simulink model "STDiscovery2016a"  (R2017b)
settings: Solver=FixedStepAuto  StartTime=0.0  StopTime=10  FixedStep=Abtastzeit  RelTol=1e-3
PreLoadFcn:
  | waijung.modelPreload; % Required for working with Waijung Blockset. Do not remove.
model workspace (MAT data in the model file):
  Abtastzeit = 0.01
  Servo_IN_min = 0.894
  SimulationDutyCycle = 27
undefined symbols (not defined in the file): HSEOSC, Link, LQFP176, ST, STM32F417IG
libraries: stm32f4_io_lib x15, simulink x10, simulink_extras x8, stm32f4_adc_lib x7, powerlib_meascontrol x3, stm32f4_device_config_lib x1
(part 4 of 5)

== system STDiscovery2016a/Debug/Subsystem2 ==
  In1 : Inport
  In2 : Inport  Port=2
  In3 : Inport  Port=3
  Enable : EnablePort
  Data Type Conversion : DataTypeConversion
  Data Type Conversion1 : DataTypeConversion
  Data Type Conversion2 : DataTypeConversion
  UART Tx : S-Function  Priority=1  FunctionName=stm32f4_usart  Parameters=configuration,uartmodule,transfer,baudrate,inputtype,outputtype,confstr,binheaderarray,binterminatorarray,asciiheader,asciiterminator,bindatalength,packetmode,varname,sampletime,sampletimestr,blockid  SFunctionDeploymentMode=off  EnableBusSupport=off  mask(stm32f4_usart){configuration=Tx, uartmodule=3, baudrate=115200, databits=8, parity=No, stopbit=1, remaptxpin=Not used, remaprxpin=Not used, flowcontrol=None, remapctspin=Not used, remaprtspin=Not used, advanceoptions=off, rxbuffersize=512, txbuffersize=512, transfer=Blocking, packetmode=Ascii, binheader='7E 7E', binterminator='03 03', porttype_double=1, porttype_single=0, porttype_int8=1, porttype_uint8=0, porttype_int16=0, porttype_uint16=0, porttype_int32=0, porttype_uint32=0, asciiformat='READ Servo:%f sec, %f Prozent, %f Hz\n', rx_asciiterminator=CRLF (0x0D 0x0A - "\r\n"), tx_asciiterminator=CRLF (0x0D 0x0A - "\r\n"), storagename=S, varname=, inputtype=[3  1 1 1], outputtype=[0], binheaderarray=[0], binterminatorarray=[0], bindatalength=0, asciiheader='READ Servo:%f sec, %f Prozent, %f Hz\n\r\n', asciiterminator=[2 13 10], sampletime=0.1, sampletimestr=-1, blockid=DebugSubsystem2UARTTx, confstr=[ "dummy", "0", "*", "*", "0", "*", "*", "0", "*", "*", "0", "*", "*", "1", "4", "3", "1", "4", "1", "512", "512", "1", "3", "115200", "8", "No", "1", "None", "USART3"], lastmodule=1}
      mask prompts: uartmodule "UART Module"; baudrate "Baud rate (bps)"; databits "Data bits"; stopbit "Stop bit"; remaptxpin "Tx Pin"; remaprxpin "Rx Pin"; flowcontrol "Hardware flow control"; remapctspin "HW Flow control, CTS Pin"; remaprtspin "HW Flow control, RTS Pin"; advanceoptions "Advance options"; rxbuffersize "Rx buffer size (bytes)"; txbuffersize "Tx buffer size (bytes)"; packetmode "Packet mode"; binheader "Binary header (example: '7E 7E')"; binterminator "Binary terminator (example: '03 03')"; porttype_double "Number of data port, type DOUBLE"; porttype_single "Number of data port, type SINGLE"; porttype_int8 "Number of data port, type INT8"; porttype_uint8 "Number of data port, type UINT8"; porttype_int16 "Number of data port, type INT16"; porttype_uint16 "Number of data port, type UINT16"; porttype_int32 "Number of data port, type INT32"; porttype_uint32 "Number of data port, type UINT32"; asciiformat "Ascii format"; rx_asciiterminator "End of packet"; tx_asciiterminator "End of packet"; storagename "Buffer"; varname "Var name"; inputtype "Input data type"; outputtype "Output data type"; binheaderarray "Binary header"; binterminatorarray "Binary terminator"; bindatalength "Binary data length"; asciiheader "Ascii header (printf format)"; asciiterminator "Ascii terminator"; sampletime "Sample time (sec)"; sampletimestr "Compiled sample time (sec) in string"; confstr "Configuration string"; lastmodule "Last module selected"
      mask help:
      | Data type for Ascii format
      | %u, %i, %d, %o, %x: uint32
      | %e, %g, %f: single
      | %c: int8
      mask init:
      | stm32f4_usart_callback('init');
      mask Help: web(fullfile(waijungdocroot,'stm32f4_usart_tx.htm'), '-browser')
      mask TypeOptions configuration: Setup | Tx | Rx
      mask Callback configuration: stm32f4_usart_callback('configuration');
      mask TypeOptions uartmodule: 1 | 2 | 3 | 4 | 5 | 6
      mask Callback uartmodule: stm32f4_usart_callback('uartmodule');
      mask Callback baudrate: stm32f4_usart_callback('baudrate');
      mask TypeOptions databits: 8
      mask TypeOptions parity: No | Odd | Even
      mask TypeOptions stopbit: 0.5 | 1 | 1.5 | 2
      mask TypeOptions remaptxpin: Not used | A9 | B6
      mask TypeOptions remaprxpin: Not used | A10 | B7
      mask TypeOptions flowcontrol: None | RTS | CTS | RTS/CTS
      mask Callback flowcontrol: stm32f4_usart_callback('flowcontrol');
      mask TypeOptions remapctspin: Not used | A11
      mask TypeOptions remaprtspin: Not used | A12
      mask Callback advanceoptions: stm32f4_usart_callback('advanceoptions');
      mask TypeOptions rxbuffersize: 16 | 32 | 64 | 128 | 256 | 512 | 1024 | 2048
      mask TypeOptions txbuffersize: 16 | 32 | 64 | 128 | 256 | 512 | 1024 | 2048
      mask TypeOptions transfer: Blocking | Non-Blocking
      mask Callback transfer: stm32f4_usart_callback('transfer');
      mask TypeOptions packetmode: Ascii | Binary | String Buffer
      mask Callback packetmode: stm32f4_usart_callback('packetmode');
      mask Callback binheader: stm32f4_usart_callback('binheader');
      mask Callback binterminator: stm32f4_usart_callback('binterminator');
      mask Callback porttype_double: stm32f4_usart_callback('porttype');
      mask Callback porttype_single: stm32f4_usart_callback('porttype');
      mask Callback porttype_int8: stm32f4_usart_callback('porttype');
      mask Callback porttype_uint8: stm32f4_usart_callback('porttype');
      mask Callback porttype_int16: stm32f4_usart_callback('porttype');
      mask Callback porttype_uint16: stm32f4_usart_callback('porttype');
      mask Callback porttype_int32: stm32f4_usart_callback('porttype');
      mask Callback porttype_uint32: stm32f4_usart_callback('porttype');
      mask Callback asciiformat: stm32f4_usart_callback('asciiformat');
      mask TypeOptions rx_asciiterminator: CR (0x0D - "\r") | LF (0x0A - "\n") | CRLF (0x0D 0x0A - "\r\n")
      mask Callback rx_asciiterminator: stm32f4_usart_callback('rx_asciiterminator');
      mask TypeOptions tx_asciiterminator: CR (0x0D - "\r") | LF (0x0A - "\n") | CRLF (0x0D 0x0A - "\r\n") | None
      mask Callback tx_asciiterminator: stm32f4_usart_callback('tx_asciiterminator');
      mask TypeOptions storagename: <Please insert a storage name> | S
      mask Callback storagename: stm32f4_usart_callback('storagename');
      mask Callback varname: stm32f4_usart_callback('varname');
      mask Callback sampletime: stm32f4_usart_callback('sampletime');
      mask Callback sampletimestr: stm32f4_usart_callback('sampletimestr');
      mask Callback blockid: stm32f4_usart_callback('blockid');
      mask Display: text(0.95, 0.5, 'Module: USART3_Tx\nPacket: Ascii\nTransfer: Blocking\nTs (sec): -1','ver','middle','hor','right'); port_label('input', 1,'single'); port_label('input', 2,'single'); port_label('input', 3,'single');
  wires:
  Data Type Conversion/1 -> UART Tx/1
  In1/1 -> Data Type Conversion/1
  In3/1 -> Data Type Conversion2/1
  In2/1 -> Data Type Conversion1/1
  Data Type Conversion1/1 -> UART Tx/2
  Data Type Conversion2/1 -> UART Tx/3

== system STDiscovery2016a/Debug/Subsystem3 ==
  In1 : Inport
  In2 : Inport  Port=2
  In3 : Inport  Port=3
  Enable : EnablePort
  Data Type Conversion : DataTypeConversion
  Data Type Conversion1 : DataTypeConversion
  Data Type Conversion2 : DataTypeConversion
  UART Tx1 : S-Function  Priority=1  FunctionName=stm32f4_usart  Parameters=configuration,uartmodule,transfer,baudrate,inputtype,outputtype,confstr,binheaderarray,binterminatorarray,asciiheader,asciiterminator,bindatalength,packetmode,varname,sampletime,sampletimestr,blockid  SFunctionDeploymentMode=off  EnableBusSupport=off  mask(stm32f4_usart){configuration=Tx, uartmodule=3, baudrate=115200, databits=8, parity=No, stopbit=1, remaptxpin=Not used, remaprxpin=Not used, flowcontrol=None, remapctspin=Not used, remaprtspin=Not used, advanceoptions=off, rxbuffersize=512, txbuffersize=512, transfer=Blocking, packetmode=Ascii, binheader='7E 7E', binterminator='03 03', porttype_double=1, porttype_single=0, porttype_int8=1, porttype_uint8=0, porttype_int16=0, porttype_uint16=0, porttype_int32=0, porttype_uint32=0, asciiformat='Antwort von ST:    TEST1: %f   , TEST2: %f   ,TEST2:  %f', rx_asciiterminator=CRLF (0x0D 0x0A - "\r\n"), tx_asciiterminator=CRLF (0x0D 0x0A - "\r\n"), storagename=S, varname=, inputtype=[3  1 1 1], outputtype=[0], binheaderarray=[0], binterminatorarray=[0], bindatalength=0, asciiheader='Antwort von ST:    TEST1: %f   , TEST2: %f   ,TEST2:  %f\r\n', asciiterminator=[2 13 10], sampletime=0.1, sampletimestr=0.1, blockid=DebugSubsystem3UARTTx1, confstr=[ "dummy", "0", "*", "*", "0", "*", "*", "0", "*", "*", "0", "*", "*", "1", "4", "3", "1", "4", "1", "512", "512", "1", "3", "115200", "8", "No", "1", "None", "USART3"], lastmodule=1}
      mask prompts: uartmodule "UART Module"; baudrate "Baud rate (bps)"; databits "Data bits"; stopbit "Stop bit"; remaptxpin "Tx Pin"; remaprxpin "Rx Pin"; flowcontrol "Hardware flow control"; remapctspin "HW Flow control, CTS Pin"; remaprtspin "HW Flow control, RTS Pin"; advanceoptions "Advance options"; rxbuffersize "Rx buffer size (bytes)"; txbuffersize "Tx buffer size (bytes)"; packetmode "Packet mode"; binheader "Binary header (example: '7E 7E')"; binterminator "Binary terminator (example: '03 03')"; porttype_double "Number of data port, type DOUBLE"; porttype_single "Number of data port, type SINGLE"; porttype_int8 "Number of data port, type INT8"; porttype_uint8 "Number of data port, type UINT8"; porttype_int16 "Number of data port, type INT16"; porttype_uint16 "Number of data port, type UINT16"; porttype_int32 "Number of data port, type INT32"; porttype_uint32 "Number of data port, type UINT32"; asciiformat "Ascii format"; rx_asciiterminator "End of packet"; tx_asciiterminator "End of packet"; storagename "Buffer"; varname "Var name"; inputtype "Input data type"; outputtype "Output data type"; binheaderarray "Binary header"; binterminatorarray "Binary terminator"; bindatalength "Binary data length"; asciiheader "Ascii header (printf format)"; asciiterminator "Ascii terminator"; sampletime "Sample time (sec)"; sampletimestr "Compiled sample time (sec) in string"; confstr "Configuration string"; lastmodule "Last module selected"
      mask help:
      | Data type for Ascii format
      | %u, %i, %d, %o, %x: uint32
      | %e, %g, %f: single
      | %c: int8
      mask init:
      | stm32f4_usart_callback('init');
      mask Help: web(fullfile(waijungdocroot,'stm32f4_usart_tx.htm'), '-browser')
      mask TypeOptions configuration: Setup | Tx | Rx
      mask Callback configuration: stm32f4_usart_callback('configuration');
      mask TypeOptions uartmodule: 1 | 2 | 3 | 4 | 5 | 6
      mask Callback uartmodule: stm32f4_usart_callback('uartmodule');
      mask Callback baudrate: stm32f4_usart_callback('baudrate');
      mask TypeOptions databits: 8
      mask TypeOptions parity: No | Odd | Even
      mask TypeOptions stopbit: 0.5 | 1 | 1.5 | 2
      mask TypeOptions remaptxpin: Not used | A9 | B6
      mask TypeOptions remaprxpin: Not used | A10 | B7
      mask TypeOptions flowcontrol: None | RTS | CTS | RTS/CTS
      mask Callback flowcontrol: stm32f4_usart_callback('flowcontrol');
      mask TypeOptions remapctspin: Not used | A11
      mask TypeOptions remaprtspin: Not used | A12
      mask Callback advanceoptions: stm32f4_usart_callback('advanceoptions');
      mask TypeOptions rxbuffersize: 16 | 32 | 64 | 128 | 256 | 512 | 1024 | 2048
      mask TypeOptions txbuffersize: 16 | 32 | 64 | 128 | 256 | 512 | 1024 | 2048
      mask TypeOptions transfer: Blocking | Non-Blocking
      mask Callback transfer: stm32f4_usart_callback('transfer');
      mask TypeOptions packetmode: Ascii | Binary | String Buffer
      mask Callback packetmode: stm32f4_usart_callback('packetmode');
      mask Callback binheader: stm32f4_usart_callback('binheader');
      mask Callback binterminator: stm32f4_usart_callback('binterminator');
      mask Callback porttype_double: stm32f4_usart_callback('porttype');
      mask Callback porttype_single: stm32f4_usart_callback('porttype');
      mask Callback porttype_int8: stm32f4_usart_callback('porttype');
      mask Callback porttype_uint8: stm32f4_usart_callback('porttype');
      mask Callback porttype_int16: stm32f4_usart_callback('porttype');
      mask Callback porttype_uint16: stm32f4_usart_callback('porttype');
      mask Callback porttype_int32: stm32f4_usart_callback('porttype');
      mask Callback porttype_uint32: stm32f4_usart_callback('porttype');
      mask Callback asciiformat: stm32f4_usart_callback('asciiformat');
      mask TypeOptions rx_asciiterminator: CR (0x0D - "\r") | LF (0x0A - "\n") | CRLF (0x0D 0x0A - "\r\n")
      mask Callback rx_asciiterminator: stm32f4_usart_callback('rx_asciiterminator');
      mask TypeOptions tx_asciiterminator: CR (0x0D - "\r") | LF (0x0A - "\n") | CRLF (0x0D 0x0A - "\r\n") | None
      mask Callback tx_asciiterminator: stm32f4_usart_callback('tx_asciiterminator');
      mask TypeOptions storagename: <Please insert a storage name> | S
      mask Callback storagename: stm32f4_usart_callback('storagename');
      mask Callback varname: stm32f4_usart_callback('varname');
      mask Callback sampletime: stm32f4_usart_callback('sampletime');
      mask Callback sampletimestr: stm32f4_usart_callback('sampletimestr');
      mask Callback blockid: stm32f4_usart_callback('blockid');
      mask Display: text(0.95, 0.5, 'Module: USART3_Tx\nPacket: Ascii\nTransfer: Blocking\nTs (sec): 0.1','ver','middle','hor','right'); port_label('input', 1,'single'); port_label('input', 2,'single'); port_label('input', 3,'single');
  wires:
  Data Type Conversion/1 -> UART Tx1/1
  In1/1 -> Data Type Conversion/1
  Data Type Conversion2/1 -> UART Tx1/3
  Data Type Conversion1/1 -> UART Tx1/2
  In2/1 -> Data Type Conversion1/1
  In3/1 -> Data Type Conversion2/1

== system STDiscovery2016a/Power Distribution Unit/Sicherung Akku ==
  note: Analoger Eingang
      | (Stromverbrauch)
  note: Digitaler Eingang
      | Sicherung zurücksetzen
  Logical Operator1 : Logic  Operator=NOT  AllPortsSameDT=off  OutDataTypeStr=boolean
  Minimaler Wert : Constant  Value=6.6
  Restspannung Akku : stm32f4_adc_lib/Regular ADC  adcmodule=1  outputdatatype=Double  prescaler=2  prescalerstr=ADC_Prescaler_Div2  chsamplingtime=Auto  chsamplingtimestr=ADC_SampleTime_480Cycles  read_an0=off  read_an1=off  read_an2=off  read_an3=off  read_an4=off  read_an5=off  read_an6=on  read_an7=off  read_an8=off  read_an9=off  read_an10=off  read_an11=off  read_an12=off  read_an13=off  read_an14=off  read_an15=off  read_an16=off  read_an17=off  read_an18=off  pinstr=GPIO_Pin_6  usedpinarray="[0  0  0  0  0  0  1  0  0  0  0  0  0  0  0  0  0  0  0]"  usedportidarray=[0]  usedpinidarray=[6]  usedpinidcount=1  sampletime=Abtastzeit  blockid=PowerDistributionUnitSicherungAkkuRestspannungAkku  enablecustomportlabel=off  cinputportlabel=0  coutputportlabel=Out1, Out2
      settings: SourceProductName=Waijung Blockset
  Sicherung ausloesen : stm32f4_io_lib/Digital Output  use_bitband=on  port=D  speed=100  porttype=Push Pull  porttypestr=PP  use_pin0=off  use_pin1=off  use_pin2=off  use_pin3=off  use_pin4=off  use_pin5=off  use_pin6=on  use_pin7=off  use_pin8=off  use_pin9=off  use_pin10=off  use_pin11=off  use_pin12=off  use_pin13=off  use_pin14=off  use_pin15=off  pinstr=GPIO_Pin_6  usedpinarray="[0  0  0  0  0  0  1  0  0  0  0  0  0  0  0  0]"  bitbandingstr="#define PowerDistributionUnitSicherungAkkuSicherungausloesen_D6 Peripheral_BB(GPIOD->ODR, 6)  /* Output pin */"  sampletime=Abtastzeit  sampletimestr=-1  blockid=PowerDistributionUnitSicherungAkkuSicherungausloesen  enablecustomportlabel=off  globalinit=off  cinputportlabel=In1, In2  coutputportlabel=0
      settings: SourceProductName=Waijung Blockset
  Sicherung gefallen : simulink_extras/Flip Flops/S-R Flip-Flop  initial_condition=0
  Sicherung nicht wieder einschalten wenn maximaler wert noch ueberschritten ist : Logic  AllPortsSameDT=off  OutDataTypeStr=boolean
  Sicherungen Ruecksetzen (User Button 1) (Loetbruecke bei sb20 noetig laut Manual) : stm32f4_io_lib/Digital Input  port=A  speed=100  porttype=None  porttypestr=NOPULL  use_pin0=on  use_pin1=off  use_pin2=off  use_pin3=off  use_pin4=off  use_pin5=off  use_pin6=off  use_pin7=off  use_pin8=off  use_pin9=off  use_pin10=off  use_pin11=off  use_pin12=off  use_pin13=off  use_pin14=off  use_pin15=off  pinstr=GPIO_Pin_0  usedpinarray="[1  0  0  0  0  0  0  0  0  0  0  0  0  0  0  0]"  bitbandingstr="#define PowerDistributionUnitSicherungAkkuSicherungenRuecksetzenUserButton1Loetbrueckebeisb20noetiglautManual_A0 Peripheral_BB(GPIOA->IDR, 0)  /* Output pin */"  sampletime=Abtastzeit  sampletimestr=-1  blockid=PowerDistributionUnitSicherungAkkuSicherungenRuecksetzenUserButton1Loetbrueckebeisb20noetiglautManual  enablecustomportlabel=off  glabalinit=off  cinputportlabel=In1, In2  coutputportlabel=Out1, Out2
      settings: SourceProductName=Waijung Blockset
  Terminator : Terminator
  Umwandlung in Range nach 5V : Gain  Gain=5/4095  ParamDataTypeStr=double  OutDataTypeStr=double
  Wurde minimaler Wert unterschritten? : RelationalOperator  Operator=>  OutDataTypeStr=boolean  RndMeth=Nearest
  wires:
  Umwandlung in Range nach 5V/1 -> Wurde minimaler Wert unterschritten?/2
  Minimaler Wert/1 -> Wurde minimaler Wert unterschritten?/1
  Wurde minimaler Wert unterschritten?/1 -> Logical Operator1/1, Sicherung gefallen/1
  Sicherung gefallen/1 -> Sicherung ausloesen/1
  Restspannung Akku/1 -> Umwandlung in Range nach 5V/1
  Sicherungen Ruecksetzen (User Button 1) (Loetbruecke bei sb20 noetig laut Manual)/1 -> Sicherung nicht wieder einschalten wenn maximaler wert noch ueberschritten ist/2
  Sicherung nicht wieder einschalten wenn maximaler wert noch ueberschritten ist/1 -> Sicherung gefallen/2
  Logical Operator1/1 -> Sicherung nicht wieder einschalten wenn maximaler wert noch ueberschritten ist/1
  Sicherung gefallen/2 -> Terminator/1

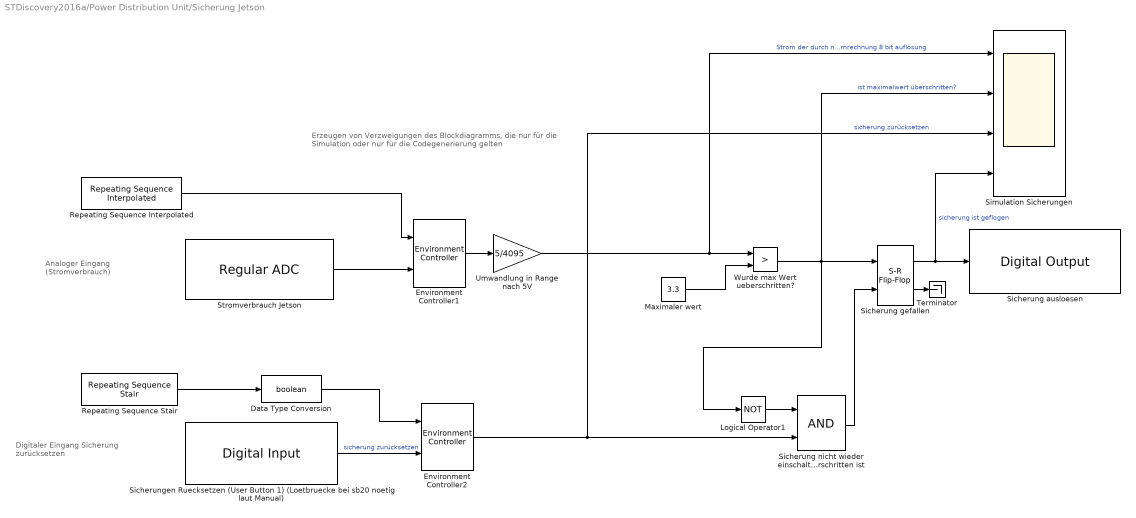
== system STDiscovery2016a/Power Distribution Unit/Sicherung Jetson ==
  note: Analoger Eingang
      | (Stromverbrauch)
  note: Erzeugen von Verzweigungen des Blockdiagramms,
      | die nur für die Simulation oder nur für die Codegenerierung gelten
  note: Digitaler Eingang
      | Sicherung zurücksetzen
  Data Type Conversion : DataTypeConversion  OutDataTypeStr=boolean
  Environment Controller1 : simulink/Signal Routing/Environment Controller
      settings: SourceProductName=Simulink  SourceProductBaseCode=SL
  Environment Controller2 : simulink/Signal Routing/Environment Controller
      settings: SourceProductName=Simulink  SourceProductBaseCode=SL
  Logical Operator1 : Logic  Operator=NOT  AllPortsSameDT=off  OutDataTypeStr=boolean
  Maximaler wert : Constant  Value=3.3
  Repeating Sequence Interpolated : simulink/Sources/Repeating Sequence Interpolated  OutValues=[2000 3000 2000].'  TimeValues=[0 5 10].'  LookUpMeth=Interpolation-Use End Values  tsamp=0.01  OutMin=[]  OutMax=[]  OutDataTypeStr=double  OutputDataTypeScalingMode=double  OutDataType=fixdt(0,8)  OutScaling=2^-10
  Repeating Sequence Stair : simulink/Sources/Repeating Sequence Stair  OutValues=[0 0 0 0 1 0 0 1 0 0].'  tsamp=1  OutMin=[]  OutMax=[]  OutDataTypeStr=double  OutputDataTypeScalingMode=double  OutDataType=fixdt(0,8)  ConRadixGroup=Best Precision: Vector-wise  OutScaling=2^-12
  Sicherung ausloesen : stm32f4_io_lib/Digital Output  use_bitband=on  port=D  speed=100  porttype=Push Pull  porttypestr=PP  use_pin0=on  use_pin1=off  use_pin2=off  use_pin3=off  use_pin4=off  use_pin5=off  use_pin6=off  use_pin7=off  use_pin8=off  use_pin9=off  use_pin10=off  use_pin11=off  use_pin12=off  use_pin13=off  use_pin14=off  use_pin15=off  pinstr=GPIO_Pin_0  usedpinarray="[1  0  0  0  0  0  0  0  0  0  0  0  0  0  0  0]"  bitbandingstr="#define PowerDistributionUnitSicherungJetsonSicherungausloesen_D0 Peripheral_BB(GPIOD->ODR, 0)  /* Output pin */"  sampletime=Abtastzeit  sampletimestr=-1  blockid=PowerDistributionUnitSicherungJetsonSicherungausloesen  enablecustomportlabel=off  globalinit=off  cinputportlabel=In1, In2  coutputportlabel=0
      settings: SourceProductName=Waijung Blockset
  Sicherung gefallen : simulink_extras/Flip Flops/S-R Flip-Flop  initial_condition=0
  Sicherung nicht wieder einschalten wenn maximaler wert noch ueberschritten ist : Logic  AllPortsSameDT=off  OutDataTypeStr=boolean
  Sicherungen Ruecksetzen (User Button 1) (Loetbruecke bei sb20 noetig laut Manual) : stm32f4_io_lib/Digital Input  port=A  speed=100  porttype=None  porttypestr=NOPULL  use_pin0=on  use_pin1=off  use_pin2=off  use_pin3=off  use_pin4=off  use_pin5=off  use_pin6=off  use_pin7=off  use_pin8=off  use_pin9=off  use_pin10=off  use_pin11=off  use_pin12=off  use_pin13=off  use_pin14=off  use_pin15=off  pinstr=GPIO_Pin_0  usedpinarray="[1  0  0  0  0  0  0  0  0  0  0  0  0  0  0  0]"  bitbandingstr="#define PowerDistributionUnitSicherungJetsonSicherungenRuecksetzenUserButton1Loetbrueckebeisb20noetiglautManual_A0 Peripheral_BB(GPIOA->IDR, 0)  /* Output pin */"  sampletime=Abtastzeit  sampletimestr=-1  blockid=PowerDistributionUnitSicherungJetsonSicherungenRuecksetzenUserButton1Loetbrueckebeisb20noetiglautManual  enablecustomportlabel=off  glabalinit=off  cinputportlabel=In1, In2  coutputportlabel=Out1, Out2
      settings: SourceProductName=Waijung Blockset
  Simulation Sicherungen : Scope  NumInputPorts=4
  Stromverbrauch Jetson : stm32f4_adc_lib/Regular ADC  adcmodule=1  outputdatatype=Double  prescaler=2  prescalerstr=ADC_Prescaler_Div2  chsamplingtime=Auto  chsamplingtimestr=ADC_SampleTime_480Cycles  read_an0=off  read_an1=on  read_an2=off  read_an3=off  read_an4=off  read_an5=off  read_an6=off  read_an7=off  read_an8=off  read_an9=off  read_an10=off  read_an11=off  read_an12=off  read_an13=off  read_an14=off  read_an15=off  read_an16=off  read_an17=off  read_an18=off  pinstr=GPIO_Pin_1  usedpinarray="[0  1  0  0  0  0  0  0  0  0  0  0  0  0  0  0  0  0  0]"  usedportidarray=[0]  usedpinidarray=[1]  usedpinidcount=1  sampletime=Abtastzeit  blockid=PowerDistributionUnitSicherungJetsonStromverbrauchJetson  enablecustomportlabel=off  cinputportlabel=0  coutputportlabel=Out1, Out2
      settings: SourceProductName=Waijung Blockset
  Terminator : Terminator
  Umwandlung in Range nach 5V : Gain  Gain=5/4095  ParamDataTypeStr=double  OutDataTypeStr=double
  Wurde max Wert ueberschritten? : RelationalOperator  Operator=>  OutDataTypeStr=boolean  RndMeth=Nearest
  wires:
  Umwandlung in Range nach 5V/1 -> Simulation Sicherungen/1, Wurde max Wert ueberschritten?/1  "Strom der durch ne spannujng ausgedrückt wird nach der umrechnung 8 bit auflösung"
  Maximaler wert/1 -> Wurde max Wert ueberschritten?/2
  Wurde max Wert ueberschritten?/1 -> Logical Operator1/1, Simulation Sicherungen/2, Sicherung gefallen/1  "ist maximalwert überschritten?"
  Environment Controller2/1 -> Sicherung nicht wieder einschalten wenn maximaler wert noch ueberschritten ist/2, Simulation Sicherungen/3  "sicherung zurücksetzen"
  Sicherung gefallen/1 -> Simulation Sicherungen/4, Sicherung ausloesen/1  "sicherung ist geflogen"
  Stromverbrauch Jetson/1 -> Environment Controller1/2
  Repeating Sequence Stair/1 -> Data Type Conversion/1
  Repeating Sequence Interpolated/1 -> Environment Controller1/1
  Sicherung nicht wieder einschalten wenn maximaler wert noch ueberschritten ist/1 -> Sicherung gefallen/2
  Logical Operator1/1 -> Sicherung nicht wieder einschalten wenn maximaler wert noch ueberschritten ist/1
  Data Type Conversion/1 -> Environment Controller2/1
  Environment Controller1/1 -> Umwandlung in Range nach 5V/1
  Sicherungen Ruecksetzen (User Button 1) (Loetbruecke bei sb20 noetig laut Manual)/1 -> Environment Controller2/2  "sicherung zurücksetzen"
  Sicherung gefallen/2 -> Terminator/1

== system STDiscovery2016a/Power Distribution Unit/Sicherung Motor ==
  note: Analoger Eingang
      | (Stromverbrauch)
  note: Digitaler Eingang
      | Sicherung zurücksetzen
  Logical Operator1 : Logic  Operator=NOT  AllPortsSameDT=off  OutDataTypeStr=boolean
  Maximaler wert : Constant  Value=3.3
  Sicherung ausloesen : stm32f4_io_lib/Digital Output  use_bitband=on  port=D  speed=100  porttype=Push Pull  porttypestr=PP  use_pin0=off  use_pin1=off  use_pin2=off  use_pin3=on  use_pin4=off  use_pin5=off  use_pin6=off  use_pin7=off  use_pin8=off  use_pin9=off  use_pin10=off  use_pin11=off  use_pin12=off  use_pin13=off  use_pin14=off  use_pin15=off  pinstr=GPIO_Pin_3  usedpinarray="[0  0  0  1  0  0  0  0  0  0  0  0  0  0  0  0]"  bitbandingstr="#define PowerDistributionUnitSicherungMotorSicherungausloesen_D3 Peripheral_BB(GPIOD->ODR, 3)  /* Output pin */"  sampletime=Abtastzeit  sampletimestr=-1  blockid=PowerDistributionUnitSicherungMotorSicherungausloesen  enablecustomportlabel=off  globalinit=off  cinputportlabel=In1, In2  coutputportlabel=0
      settings: SourceProductName=Waijung Blockset
  Sicherung gefallen : simulink_extras/Flip Flops/S-R Flip-Flop  initial_condition=0
  Sicherung nicht wieder einschalten wenn maximaler wert noch ueberschritten ist : Logic  AllPortsSameDT=off  OutDataTypeStr=boolean
  Sicherungen Ruecksetzen (User Button 1) (Loetbruecke bei sb20 noetig laut Manual) : stm32f4_io_lib/Digital Input  port=A  speed=100  porttype=None  porttypestr=NOPULL  use_pin0=on  use_pin1=off  use_pin2=off  use_pin3=off  use_pin4=off  use_pin5=off  use_pin6=off  use_pin7=off  use_pin8=off  use_pin9=off  use_pin10=off  use_pin11=off  use_pin12=off  use_pin13=off  use_pin14=off  use_pin15=off  pinstr=GPIO_Pin_0  usedpinarray="[1  0  0  0  0  0  0  0  0  0  0  0  0  0  0  0]"  bitbandingstr="#define PowerDistributionUnitSicherungMotorSicherungenRuecksetzenUserButton1Loetbrueckebeisb20noetiglautManual_A0 Peripheral_BB(GPIOA->IDR, 0)  /* Output pin */"  sampletime=Abtastzeit  sampletimestr=-1  blockid=PowerDistributionUnitSicherungMotorSicherungenRuecksetzenUserButton1Loetbrueckebeisb20noetiglautManual  enablecustomportlabel=off  glabalinit=off  cinputportlabel=In1, In2  coutputportlabel=Out1, Out2
      settings: SourceProductName=Waijung Blockset
  Stromverbrauch Motor : stm32f4_adc_lib/Regular ADC  adcmodule=1  outputdatatype=Double  prescaler=2  prescalerstr=ADC_Prescaler_Div2  chsamplingtime=Auto  chsamplingtimestr=ADC_SampleTime_480Cycles  read_an0=off  read_an1=off  read_an2=off  read_an3=on  read_an4=off  read_an5=off  read_an6=off  read_an7=off  read_an8=off  read_an9=off  read_an10=off  read_an11=off  read_an12=off  read_an13=off  read_an14=off  read_an15=off  read_an16=off  read_an17=off  read_an18=off  pinstr=GPIO_Pin_3  usedpinarray="[0  0  0  1  0  0  0  0  0  0  0  0  0  0  0  0  0  0  0]"  usedportidarray=[0]  usedpinidarray=[3]  usedpinidcount=1  sampletime=Abtastzeit  blockid=PowerDistributionUnitSicherungMotorStromverbrauchMotor  enablecustomportlabel=off  cinputportlabel=0  coutputportlabel=Out1, Out2
      settings: SourceProductName=Waijung Blockset
  Terminator : Terminator
  Umwandlung in Range nach 5V : Gain  Gain=5/4095  ParamDataTypeStr=double  OutDataTypeStr=double
  Wurde max Wert überschritten? : RelationalOperator  Operator=>  OutDataTypeStr=boolean  RndMeth=Nearest
  wires:
  Umwandlung in Range nach 5V/1 -> Wurde max Wert überschritten?/1
  Maximaler wert/1 -> Wurde max Wert überschritten?/2
  Wurde max Wert überschritten?/1 -> Logical Operator1/1, Sicherung gefallen/1
  Sicherung gefallen/1 -> Sicherung ausloesen/1
  Stromverbrauch Motor/1 -> Umwandlung in Range nach 5V/1
  Sicherungen Ruecksetzen (User Button 1) (Loetbruecke bei sb20 noetig laut Manual)/1 -> Sicherung nicht wieder einschalten wenn maximaler wert noch ueberschritten ist/2
  Sicherung nicht wieder einschalten wenn maximaler wert noch ueberschritten ist/1 -> Sicherung gefallen/2
  Logical Operator1/1 -> Sicherung nicht wieder einschalten wenn maximaler wert noch ueberschritten ist/1
  Sicherung gefallen/2 -> Terminator/1

== system STDiscovery2016a/Power Distribution Unit/Sicherung Reciever ==
  note: Analoger Eingang
      | (Stromverbrauch)
  note: Digitaler Eingang
      | Sicherung zurücksetzen
  Logical Operator1 : Logic  Operator=NOT  AllPortsSameDT=off  OutDataTypeStr=boolean
  Maximaler wert : Constant  Value=3.3
  Sicherung ausloesen : stm32f4_io_lib/Digital Output  use_bitband=on  port=D  speed=100  porttype=Push Pull  porttypestr=PP  use_pin0=off  use_pin1=off  use_pin2=off  use_pin3=off  use_pin4=off  use_pin5=on  use_pin6=off  use_pin7=off  use_pin8=off  use_pin9=off  use_pin10=off  use_pin11=off  use_pin12=off  use_pin13=off  use_pin14=off  use_pin15=off  pinstr=GPIO_Pin_5  usedpinarray="[0  0  0  0  0  1  0  0  0  0  0  0  0  0  0  0]"  bitbandingstr="#define PowerDistributionUnitSicherungRecieverSicherungausloesen_D5 Peripheral_BB(GPIOD->ODR, 5)  /* Output pin */"  sampletime=Abtastzeit  sampletimestr=-1  blockid=PowerDistributionUnitSicherungRecieverSicherungausloesen  enablecustomportlabel=off  globalinit=off  cinputportlabel=In1, In2  coutputportlabel=0
      settings: SourceProductName=Waijung Blockset
  Sicherung gefallen : simulink_extras/Flip Flops/S-R Flip-Flop  initial_condition=0
  Sicherung nicht wieder einschalten wenn maximaler wert noch ueberschritten ist : Logic  AllPortsSameDT=off  OutDataTypeStr=boolean
  Sicherungen Ruecksetzen (User Button 1) (Loetbruecke bei sb20 noetig laut Manual) : stm32f4_io_lib/Digital Input  port=A  speed=100  porttype=None  porttypestr=NOPULL  use_pin0=on  use_pin1=off  use_pin2=off  use_pin3=off  use_pin4=off  use_pin5=off  use_pin6=off  use_pin7=off  use_pin8=off  use_pin9=off  use_pin10=off  use_pin11=off  use_pin12=off  use_pin13=off  use_pin14=off  use_pin15=off  pinstr=GPIO_Pin_0  usedpinarray="[1  0  0  0  0  0  0  0  0  0  0  0  0  0  0  0]"  bitbandingstr="#define PowerDistributionUnitSicherungRecieverSicherungenRuecksetzenUserButton1Loetbrueckebeisb20noetiglautManual_A0 Peripheral_BB(GPIOA->IDR, 0)  /* Output pin */"  sampletime=Abtastzeit  sampletimestr=-1  blockid=PowerDistributionUnitSicherungRecieverSicherungenRuecksetzenUserButton1Loetbrueckebeisb20noetiglautManual  enablecustomportlabel=off  glabalinit=off  cinputportlabel=In1, In2  coutputportlabel=Out1, Out2
      settings: SourceProductName=Waijung Blockset
  Stromverbrauch Reciever : stm32f4_adc_lib/Regular ADC  adcmodule=1  outputdatatype=Double  prescaler=2  prescalerstr=ADC_Prescaler_Div2  chsamplingtime=Auto  chsamplingtimestr=ADC_SampleTime_480Cycles  read_an0=off  read_an1=off  read_an2=off  read_an3=off  read_an4=off  read_an5=on  read_an6=off  read_an7=off  read_an8=off  read_an9=off  read_an10=off  read_an11=off  read_an12=off  read_an13=off  read_an14=off  read_an15=off  read_an16=off  read_an17=off  read_an18=off  pinstr=GPIO_Pin_5  usedpinarray="[0  0  0  0  0  1  0  0  0  0  0  0  0  0  0  0  0  0  0]"  usedportidarray=[0]  usedpinidarray=[5]  usedpinidcount=1  sampletime=Abtastzeit  blockid=PowerDistributionUnitSicherungRecieverStromverbrauchReciever  enablecustomportlabel=off  cinputportlabel=0  coutputportlabel=Out1, Out2
      settings: SourceProductName=Waijung Blockset
  Terminator : Terminator
  Umwandlung in Range nach 5V : Gain  Gain=5/4095  ParamDataTypeStr=double  OutDataTypeStr=double
  Wurde max Wert überschritten? : RelationalOperator  Operator=>  OutDataTypeStr=boolean  RndMeth=Nearest
  wires:
  Umwandlung in Range nach 5V/1 -> Wurde max Wert überschritten?/1
  Maximaler wert/1 -> Wurde max Wert überschritten?/2
  Wurde max Wert überschritten?/1 -> Logical Operator1/1, Sicherung gefallen/1
  Sicherung gefallen/1 -> Sicherung ausloesen/1
  Stromverbrauch Reciever/1 -> Umwandlung in Range nach 5V/1
  Sicherungen Ruecksetzen (User Button 1) (Loetbruecke bei sb20 noetig laut Manual)/1 -> Sicherung nicht wieder einschalten wenn maximaler wert noch ueberschritten ist/2
  Sicherung nicht wieder einschalten wenn maximaler wert noch ueberschritten ist/1 -> Sicherung gefallen/2
  Logical Operator1/1 -> Sicherung nicht wieder einschalten wenn maximaler wert noch ueberschritten ist/1
  Sicherung gefallen/2 -> Terminator/1

== system STDiscovery2016a/Power Distribution Unit/Sicherung ST ==
  note: Analoger Eingang
      | (Stromverbrauch)
  note: Digitaler Eingang
      | Sicherung zurücksetzen
  Logical Operator1 : Logic  Operator=NOT  AllPortsSameDT=off  OutDataTypeStr=boolean
  Maximaler wert : Constant  Value=3.3
  Sicherung ausloesen : stm32f4_io_lib/Digital Output  use_bitband=on  port=D  speed=100  porttype=Push Pull  porttypestr=PP  use_pin0=off  use_pin1=off  use_pin2=on  use_pin3=off  use_pin4=off  use_pin5=off  use_pin6=off  use_pin7=off  use_pin8=off  use_pin9=off  use_pin10=off  use_pin11=off  use_pin12=off  use_pin13=off  use_pin14=off  use_pin15=off  pinstr=GPIO_Pin_2  usedpinarray="[0  0  1  0  0  0  0  0  0  0  0  0  0  0  0  0]"  bitbandingstr="#define PowerDistributionUnitSicherungSTSicherungausloesen_D2 Peripheral_BB(GPIOD->ODR, 2)  /* Output pin */"  sampletime=Abtastzeit  sampletimestr=-1  blockid=PowerDistributionUnitSicherungSTSicherungausloesen  enablecustomportlabel=off  globalinit=off  cinputportlabel=In1, In2  coutputportlabel=0
      settings: SourceProductName=Waijung Blockset
  Sicherung gefallen : simulink_extras/Flip Flops/S-R Flip-Flop  initial_condition=0
  Sicherung nicht wieder einschalten wenn maximaler wert noch ueberschritten ist : Logic  AllPortsSameDT=off  OutDataTypeStr=boolean
  Sicherungen Ruecksetzen (User Button 1) (Loetbruecke bei sb20 noetig laut Manual) : stm32f4_io_lib/Digital Input  port=A  speed=100  porttype=None  porttypestr=NOPULL  use_pin0=on  use_pin1=off  use_pin2=off  use_pin3=off  use_pin4=off  use_pin5=off  use_pin6=off  use_pin7=off  use_pin8=off  use_pin9=off  use_pin10=off  use_pin11=off  use_pin12=off  use_pin13=off  use_pin14=off  use_pin15=off  pinstr=GPIO_Pin_0  usedpinarray="[1  0  0  0  0  0  0  0  0  0  0  0  0  0  0  0]"  bitbandingstr="#define PowerDistributionUnitSicherungSTSicherungenRuecksetzenUserButton1Loetbrueckebeisb20noetiglautManual_A0 Peripheral_BB(GPIOA->IDR, 0)  /* Output pin */"  sampletime=Abtastzeit  sampletimestr=-1  blockid=PowerDistributionUnitSicherungSTSicherungenRuecksetzenUserButton1Loetbrueckebeisb20noetiglautManual  enablecustomportlabel=off  glabalinit=off  cinputportlabel=In1, In2  coutputportlabel=Out1, Out2
      settings: SourceProductName=Waijung Blockset
  Stromverbrauch ST : stm32f4_adc_lib/Regular ADC  adcmodule=1  outputdatatype=Double  prescaler=2  prescalerstr=ADC_Prescaler_Div2  chsamplingtime=Auto  chsamplingtimestr=ADC_SampleTime_480Cycles  read_an0=off  read_an1=off  read_an2=on  read_an3=off  read_an4=off  read_an5=off  read_an6=off  read_an7=off  read_an8=off  read_an9=off  read_an10=off  read_an11=off  read_an12=off  read_an13=off  read_an14=off  read_an15=off  read_an16=off  read_an17=off  read_an18=off  pinstr=GPIO_Pin_2  usedpinarray="[0  0  1  0  0  0  0  0  0  0  0  0  0  0  0  0  0  0  0]"  usedportidarray=[0]  usedpinidarray=[2]  usedpinidcount=1  sampletime=Abtastzeit  blockid=PowerDistributionUnitSicherungSTStromverbrauchST  enablecustomportlabel=on  cinputportlabel=0  coutputportlabel=Out1, Out2
      settings: SourceProductName=Waijung Blockset
  Terminator : Terminator
  Umwandlung in Range nach 5V : Gain  Gain=5/4095  ParamDataTypeStr=double  OutDataTypeStr=double
  Wurde max Wert überschritten? : RelationalOperator  Operator=>  OutDataTypeStr=boolean  RndMeth=Nearest
  wires:
  Umwandlung in Range nach 5V/1 -> Wurde max Wert überschritten?/1  "Strom der durch ne spannujng ausgedrückt wird nach der umrechnung 8 bit auflösung"
  Maximaler wert/1 -> Wurde max Wert überschritten?/2
  Wurde max Wert überschritten?/1 -> Logical Operator1/1, Sicherung gefallen/1  "ist maximalwert überschritten?"
  Sicherung gefallen/1 -> Sicherung ausloesen/1  "sicherung ist geflogen"
  Stromverbrauch ST/1 -> Umwandlung in Range nach 5V/1
  Sicherungen Ruecksetzen (User Button 1) (Loetbruecke bei sb20 noetig laut Manual)/1 -> Sicherung nicht wieder einschalten wenn maximaler wert noch ueberschritten ist/2
  Sicherung nicht wieder einschalten wenn maximaler wert noch ueberschritten ist/1 -> Sicherung gefallen/2
  Logical Operator1/1 -> Sicherung nicht wieder einschalten wenn maximaler wert noch ueberschritten ist/1
  Sicherung gefallen/2 -> Terminator/1

== system STDiscovery2016a/Power Distribution Unit/Sicherung Servo ==
  note: Analoger Eingang
      | (Stromverbrauch)
  note: Digitaler Eingang
      | Sicherung zurücksetzen
  Logical Operator1 : Logic  Operator=NOT  AllPortsSameDT=off  OutDataTypeStr=boolean
  Maximaler wert : Constant  Value=3.3
  Sicherung ausloesen : stm32f4_io_lib/Digital Output  use_bitband=on  port=D  speed=100  porttype=Push Pull  porttypestr=PP  use_pin0=off  use_pin1=off  use_pin2=off  use_pin3=off  use_pin4=on  use_pin5=off  use_pin6=off  use_pin7=off  use_pin8=off  use_pin9=off  use_pin10=off  use_pin11=off  use_pin12=off  use_pin13=off  use_pin14=off  use_pin15=off  pinstr=GPIO_Pin_4  usedpinarray="[0  0  0  0  1  0  0  0  0  0  0  0  0  0  0  0]"  bitbandingstr="#define PowerDistributionUnitSicherungServoSicherungausloesen_D4 Peripheral_BB(GPIOD->ODR, 4)  /* Output pin */"  sampletime=Abtastzeit  sampletimestr=-1  blockid=PowerDistributionUnitSicherungServoSicherungausloesen  enablecustomportlabel=off  globalinit=off  cinputportlabel=In1, In2  coutputportlabel=0
      settings: SourceProductName=Waijung Blockset
  Sicherung gefallen : simulink_extras/Flip Flops/S-R Flip-Flop  initial_condition=0
  Sicherung nicht wieder einschalten wenn maximaler wert noch ueberschritten ist : Logic  AllPortsSameDT=off  OutDataTypeStr=boolean
  Sicherungen Ruecksetzen (User Button 1) (Loetbruecke bei sb20 noetig laut Manual) : stm32f4_io_lib/Digital Input  port=A  speed=100  porttype=None  porttypestr=NOPULL  use_pin0=on  use_pin1=off  use_pin2=off  use_pin3=off  use_pin4=off  use_pin5=off  use_pin6=off  use_pin7=off  use_pin8=off  use_pin9=off  use_pin10=off  use_pin11=off  use_pin12=off  use_pin13=off  use_pin14=off  use_pin15=off  pinstr=GPIO_Pin_0  usedpinarray="[1  0  0  0  0  0  0  0  0  0  0  0  0  0  0  0]"  bitbandingstr="#define PowerDistributionUnitSicherungServoSicherungenRuecksetzenUserButton1Loetbrueckebeisb20noetiglautManual_A0 Peripheral_BB(GPIOA->IDR, 0)  /* Output pin */"  sampletime=Abtastzeit  sampletimestr=-1  blockid=PowerDistributionUnitSicherungServoSicherungenRuecksetzenUserButton1Loetbrueckebeisb20noetiglautManual  enablecustomportlabel=off  glabalinit=off  cinputportlabel=In1, In2  coutputportlabel=Out1, Out2
      settings: SourceProductName=Waijung Blockset
  Stromverbrauch Servo : stm32f4_adc_lib/Regular ADC  adcmodule=1  outputdatatype=Double  prescaler=2  prescalerstr=ADC_Prescaler_Div2  chsamplingtime=Auto  chsamplingtimestr=ADC_SampleTime_480Cycles  read_an0=off  read_an1=off  read_an2=off  read_an3=off  read_an4=on  read_an5=off  read_an6=off  read_an7=off  read_an8=off  read_an9=off  read_an10=off  read_an11=off  read_an12=off  read_an13=off  read_an14=off  read_an15=off  read_an16=off  read_an17=off  read_an18=off  pinstr=GPIO_Pin_4  usedpinarray="[0  0  0  0  1  0  0  0  0  0  0  0  0  0  0  0  0  0  0]"  usedportidarray=[0]  usedpinidarray=[4]  usedpinidcount=1  sampletime=Abtastzeit  blockid=PowerDistributionUnitSicherungServoStromverbrauchServo  enablecustomportlabel=off  cinputportlabel=0  coutputportlabel=Out1, Out2
      settings: SourceProductName=Waijung Blockset
  Terminator : Terminator
  Umwandlung in Range nach 5V : Gain  Gain=5/4095  ParamDataTypeStr=double  OutDataTypeStr=double
  Wurde max Wert überschritten? : RelationalOperator  Operator=>  OutDataTypeStr=boolean  RndMeth=Nearest
  wires:
  Umwandlung in Range nach 5V/1 -> Wurde max Wert überschritten?/1
  Maximaler wert/1 -> Wurde max Wert überschritten?/2
  Wurde max Wert überschritten?/1 -> Logical Operator1/1, Sicherung gefallen/1
  Sicherung gefallen/1 -> Sicherung ausloesen/1
  Stromverbrauch Servo/1 -> Umwandlung in Range nach 5V/1
  Sicherungen Ruecksetzen (User Button 1) (Loetbruecke bei sb20 noetig laut Manual)/1 -> Sicherung nicht wieder einschalten wenn maximaler wert noch ueberschritten ist/2
  Sicherung nicht wieder einschalten wenn maximaler wert noch ueberschritten ist/1 -> Sicherung gefallen/2
  Logical Operator1/1 -> Sicherung nicht wieder einschalten wenn maximaler wert noch ueberschritten ist/1
  Sicherung gefallen/2 -> Terminator/1

== system STDiscovery2016a/Power Distribution Unit/Sicherung Spare ==
  note: Analoger Eingang
      | (Stromverbrauch)
  note: Digitaler Eingang
      | Sicherung zurücksetzen
  Logical Operator1 : Logic  Operator=NOT  AllPortsSameDT=off  OutDataTypeStr=boolean
  Minimaler Wert : Constant  Value=6.6
  Restspannung Akku : stm32f4_adc_lib/Regular ADC  adcmodule=1  outputdatatype=Double  prescaler=2  prescalerstr=ADC_Prescaler_Div2  chsamplingtime=Auto  chsamplingtimestr=ADC_SampleTime_480Cycles  read_an0=off  read_an1=off  read_an2=off  read_an3=off  read_an4=off  read_an5=off  read_an6=off  read_an7=on  read_an8=off  read_an9=off  read_an10=off  read_an11=off  read_an12=off  read_an13=off  read_an14=off  read_an15=off  read_an16=off  read_an17=off  read_an18=off  pinstr=GPIO_Pin_7  usedpinarray="[0  0  0  0  0  0  0  1  0  0  0  0  0  0  0  0  0  0  0]"  usedportidarray=[0]  usedpinidarray=[7]  usedpinidcount=1  sampletime=Abtastzeit  blockid=PowerDistributionUnitSicherungSpareRestspannungAkku  enablecustomportlabel=off  cinputportlabel=0  coutputportlabel=Out1, Out2
      settings: SourceProductName=Waijung Blockset
  Sicherung ausloesen : stm32f4_io_lib/Digital Output  use_bitband=on  port=D  speed=100  porttype=Push Pull  porttypestr=PP  use_pin0=off  use_pin1=off  use_pin2=off  use_pin3=off  use_pin4=off  use_pin5=off  use_pin6=off  use_pin7=on  use_pin8=off  use_pin9=off  use_pin10=off  use_pin11=off  use_pin12=off  use_pin13=off  use_pin14=off  use_pin15=off  pinstr=GPIO_Pin_7  usedpinarray="[0  0  0  0  0  0  0  1  0  0  0  0  0  0  0  0]"  bitbandingstr="#define PowerDistributionUnitSicherungSpareSicherungausloesen_D7 Peripheral_BB(GPIOD->ODR, 7)  /* Output pin */"  sampletime=Abtastzeit  sampletimestr=-1  blockid=PowerDistributionUnitSicherungSpareSicherungausloesen  enablecustomportlabel=off  globalinit=off  cinputportlabel=In1, In2  coutputportlabel=0
      settings: SourceProductName=Waijung Blockset
  Sicherung gefallen : simulink_extras/Flip Flops/S-R Flip-Flop  initial_condition=0
  Sicherung nicht wieder einschalten wenn maximaler wert noch ueberschritten ist : Logic  AllPortsSameDT=off  OutDataTypeStr=boolean
  Sicherungen Ruecksetzen (User Button 1) (Loetbruecke bei sb20 noetig laut Manual) : stm32f4_io_lib/Digital Input  port=A  speed=100  porttype=None  porttypestr=NOPULL  use_pin0=on  use_pin1=off  use_pin2=off  use_pin3=off  use_pin4=off  use_pin5=off  use_pin6=off  use_pin7=off  use_pin8=off  use_pin9=off  use_pin10=off  use_pin11=off  use_pin12=off  use_pin13=off  use_pin14=off  use_pin15=off  pinstr=GPIO_Pin_0  usedpinarray="[1  0  0  0  0  0  0  0  0  0  0  0  0  0  0  0]"  bitbandingstr="#define PowerDistributionUnitSicherungSpareSicherungenRuecksetzenUserButton1Loetbrueckebeisb20noetiglautManual_A0 Peripheral_BB(GPIOA->IDR, 0)  /* Output pin */"  sampletime=Abtastzeit  sampletimestr=-1  blockid=PowerDistributionUnitSicherungSpareSicherungenRuecksetzenUserButton1Loetbrueckebeisb20noetiglautManual  enablecustomportlabel=off  glabalinit=off  cinputportlabel=In1, In2  coutputportlabel=Out1, Out2
      settings: SourceProductName=Waijung Blockset
  Terminator : Terminator
  Umwandlung in Range nach 5V : Gain  Gain=5/4095  ParamDataTypeStr=double  OutDataTypeStr=double
  Wurde minimaler Wert unterschritten? : RelationalOperator  Operator=>  OutDataTypeStr=boolean  RndMeth=Nearest
  wires:
  Umwandlung in Range nach 5V/1 -> Wurde minimaler Wert unterschritten?/2
  Minimaler Wert/1 -> Wurde minimaler Wert unterschritten?/1
  Wurde minimaler Wert unterschritten?/1 -> Logical Operator1/1, Sicherung gefallen/1
  Sicherung gefallen/1 -> Sicherung ausloesen/1
  Restspannung Akku/1 -> Umwandlung in Range nach 5V/1
  Sicherungen Ruecksetzen (User Button 1) (Loetbruecke bei sb20 noetig laut Manual)/1 -> Sicherung nicht wieder einschalten wenn maximaler wert noch ueberschritten ist/2
  Sicherung nicht wieder einschalten wenn maximaler wert noch ueberschritten ist/1 -> Sicherung gefallen/2
  Logical Operator1/1 -> Sicherung nicht wieder einschalten wenn maximaler wert noch ueberschritten ist/1
  Sicherung gefallen/2 -> Terminator/1

== system STDiscovery2016a/Aktorik/Ansteuerung Motor/Logik  ==
  Fernbedienung Signal : Inport
  Eingriff_Fernbedienung : Inport  Port=2
  Jetson Signal : Inport  Port=3
  "Erst 1s stoppen, dann Fernbedieung" : Switch  Criteria=u2 > Threshold
  "Mittelwert, in % wenn Fernsteuerung in der Mitte steht" : Constant  Value=7.45
  Modus Auswahl : Switch  Criteria=u2 > Threshold
  Wartezeit Anhalten (Einschaltverzögerung) : powerlib_meascontrol/Logic/On Delay  DelayType=On delay  delay=1  ic=1  Ts=0
      settings: SourceProductName=Simscape Power Systems
  Output Pin : Outport
  wires:
  Fernbedienung Signal/1 -> "Erst 1s stoppen, dann Fernbedieung"/1  "manuell"
  "Erst 1s stoppen, dann Fernbedieung"/1 -> Modus Auswahl/1  "manuell"
  Modus Auswahl/1 -> Output Pin/1
  Jetson Signal/1 -> Modus Auswahl/3  "autonom"
  Eingriff_Fernbedienung/1 -> Wartezeit Anhalten (Einschaltverzögerung)/1, Modus Auswahl/2
  Wartezeit Anhalten (Einschaltverzögerung)/1 -> "Erst 1s stoppen, dann Fernbedieung"/2
  "Mittelwert, in % wenn Fernsteuerung in der Mitte steht"/1 -> "Erst 1s stoppen, dann Fernbedieung"/3

== system STDiscovery2016a/Aktorik/Ansteuerung Motor/Plausibilitäts Check ==
  In1 : Inport
  "Gib Mittelstellung aus, wenn mit Signal etwas nicht Stimmt" : Switch  Criteria=u2 > Threshold
  Logical Operator : Logic  AllPortsSameDT=off  OutDataTypeStr=boolean
  Mittelstellung : Constant  Value=0.0015
  Relational Operator : RelationalOperator  Operator=<  OutDataTypeStr=boolean  RndMeth=Nearest
  Relational Operator1 : RelationalOperator  Operator=>  OutDataTypeStr=boolean  RndMeth=Nearest
  "ok max " : Constant  Value=0.0021
  ok min : Constant  Value=0.001
  Out1 : Outport
  wires:
  In1/1 -> Relational Operator1/1, Relational Operator/1, "Gib Mittelstellung aus, wenn mit Signal etwas nicht Stimmt"/1
  Logical Operator/1 -> "Gib Mittelstellung aus, wenn mit Signal etwas nicht Stimmt"/2
  "Gib Mittelstellung aus, wenn mit Signal etwas nicht Stimmt"/1 -> Out1/1
  Mittelstellung/1 -> "Gib Mittelstellung aus, wenn mit Signal etwas nicht Stimmt"/3
  Relational Operator1/1 -> Logical Operator/2
  Relational Operator/1 -> Logical Operator/1
  ok min/1 -> Relational Operator1/2
  "ok max "/1 -> Relational Operator/2

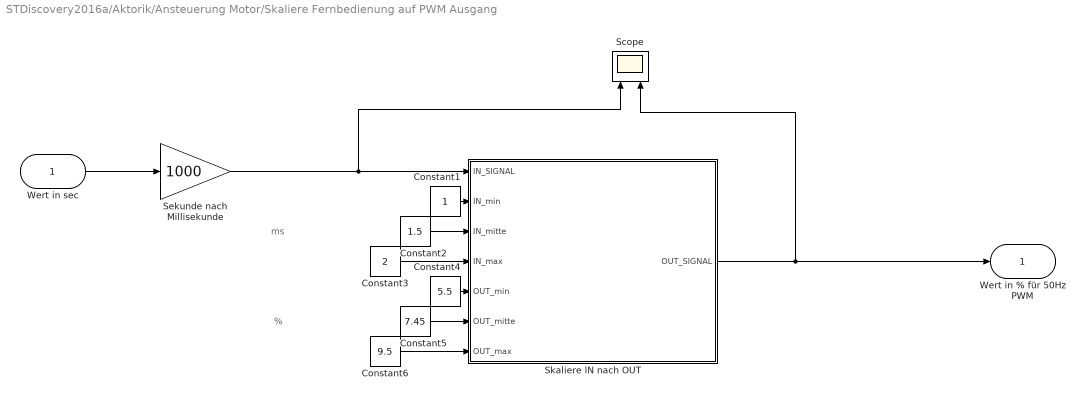
== system STDiscovery2016a/Aktorik/Ansteuerung Motor/Skaliere Fernbedienung auf PWM Ausgang ==
  note: %
  note: ms
  Wert in sec : Inport
  Constant1 : Constant
  Constant2 : Constant  Value=1.5
  Constant3 : Constant  Value=2
  Constant4 : Constant  Value=5.5
  Constant5 : Constant  Value=7.45
  Constant6 : Constant  Value=9.5
  Scope : Scope  NumInputPorts=2
  Sekunde nach Millisekunde : Gain  Gain=1000
  Skaliere lN nach OUT : Subsystem
  Wert in % für 50Hz PWM : Outport
  wires:
  Constant4/1 -> Skaliere lN nach OUT/5(OUT_min)
  Wert in sec/1 -> Sekunde nach Millisekunde/1
  Constant5/1 -> Skaliere lN nach OUT/6(OUT_mitte)
  Skaliere lN nach OUT/1(OUT_SIGNAL) -> Scope/2, Wert in % für 50Hz PWM/1
  Constant3/1 -> Skaliere lN nach OUT/4(IN_max)
  Constant2/1 -> Skaliere lN nach OUT/3(IN_mitte)
  Constant1/1 -> Skaliere lN nach OUT/2(IN_min)
  Constant6/1 -> Skaliere lN nach OUT/7(OUT_max)
  Sekunde nach Millisekunde/1 -> Scope/1, Skaliere lN nach OUT/1(IN_SIGNAL)

== system STDiscovery2016a/Aktorik/Ansteuerung Motor/Skaliere Jetson( + -100) auf PWM Ausgang ==
  note: %
  note: 100(Gas)
      | -100(Rückwärts)
  Wert in sec : Inport
  Constant1 : Constant  Value=100
  Constant2 : Constant  Value=0
  Constant3 : Constant  Value=-100
  Constant4 : Constant  Value=5.5
  Constant5 : Constant  Value=7.45
  Constant6 : Constant  Value=9.5
  Skaliere lN nach OUT : Subsystem
  Wert in % für 50Hz PWM : Outport
  wires:
  Constant4/1 -> Skaliere lN nach OUT/5(OUT_min)
  Constant5/1 -> Skaliere lN nach OUT/6(OUT_mitte)
  Skaliere lN nach OUT/1(OUT_SIGNAL) -> Wert in % für 50Hz PWM/1
  Constant3/1 -> Skaliere lN nach OUT/4(IN_max)
  Constant2/1 -> Skaliere lN nach OUT/3(IN_mitte)
  Constant1/1 -> Skaliere lN nach OUT/2(IN_min)
  Constant6/1 -> Skaliere lN nach OUT/7(OUT_max)
  Wert in sec/1 -> Skaliere lN nach OUT/1(IN_SIGNAL)
